simulink model "totalSystem_nath2"  (R2012b)
settings: Solver=ode45  StartTime=0.0  StopTime=50.0  RelTol=1e-5
libraries: simulink x1
settings Model: Creator=Labo  LastModifiedBy=nathdwek
settings DataIOCC: SignalLoggingSaveFormat=ModelDataLogs
settings OptimizationCC: ExpressionDepthLimit=128
settings DebuggingCC: MultiTaskDSMMsg=warning  MultiTaskCondExecSysMsg=none  StrictBusMsg=None
settings RTWCC: IncludeERTFirstTime=on
settings CodeAppCC: CustomSymbolStrType=$N$R$M_T  InternalIdentifier=Shortened

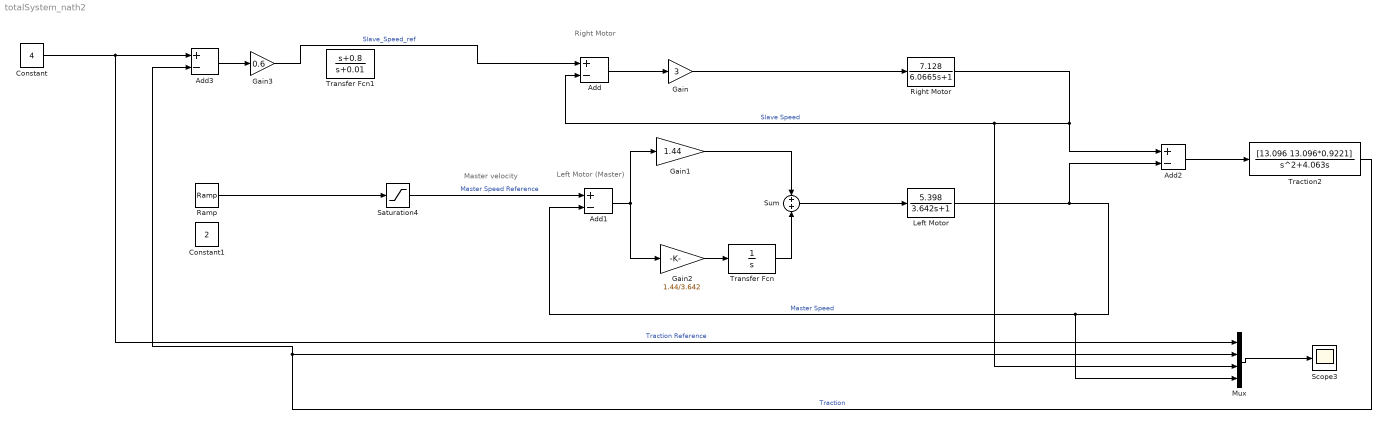
== system totalSystem_nath2 ==
  note: Master velocity
  note: Left Motor (Master)
  note: Right Motor
  Add{,1..3} (4 alike) : Sum  Inputs=+-
  Constant : Constant  Value=4
  Constant1 : Constant  Value=2
  Gain : Gain  Gain=3
  Gain1 : Gain  Gain=1.44
  Gain2 : Gain  Gain=1.44/3.642
  Gain3 : Gain  Gain=0.6
  "Left Motor " : TransferFcn  Numerator=[5.398]  Denominator=[3.642 1]  ContinuousStateAttributes='v'
  Mux : Mux
  Ramp : simulink/Sources/Ramp  slope=2/8  start=0  X0=0
  "Right Motor " : TransferFcn  Numerator=[7.128]  Denominator=[6.0665 1]  ContinuousStateAttributes='v'
  Saturation4 : Saturate  UpperLimit=2  LowerLimit=0
  Scope3 : Scope
      settings: ShowLegends=on
  Sum : Sum  Inputs=+|+
  Traction2 : TransferFcn  Numerator=[13.096 13.096*0.9221]  Denominator=[1 4.063 0]
  Transfer Fcn : TransferFcn  Denominator=[1 0]
  Transfer Fcn1 : TransferFcn  Numerator=[1 0.8]  Denominator=[1 0.01]
  wires:
  Add/1 -> Gain/1
  "Right Motor "/1 -> Add2/1, Mux/3, Add/2  "Slave Speed"
  Gain/1 -> "Right Motor "/1
  Add1/1 -> Gain2/1, Gain1/1
  "Left Motor "/1 -> Mux/4, Add1/2, Add2/2  "Master Speed"
  Sum/1 -> "Left Motor "/1
  Traction2/1 -> Add3/2, Mux/2  "Traction"
  Constant/1 -> Mux/1, Add3/1  "Traction Reference"
  Saturation4/1 -> Add1/1  "Master Speed Reference"
  Mux/1 -> Scope3/1
  Add2/1 -> Traction2/1
  Gain2/1 -> Transfer Fcn/1
  Transfer Fcn/1 -> Sum/2
  Gain1/1 -> Sum/1
  Ramp/1 -> Saturation4/1
  Add3/1 -> Gain3/1
  Gain3/1 -> Add/1  "Slave_Speed_ref"
